simulink model "sampleModel128"  (R2021b)
settings: Solver=VariableStepAuto  StartTime=0.0  StopTime=10.0  RelTol=1e-3
undefined symbols (not defined in the file or in its folder): DiscIntNeverNeededParam
libraries: simulink x5
settings Model: Creator=user  LastModifiedBy=user

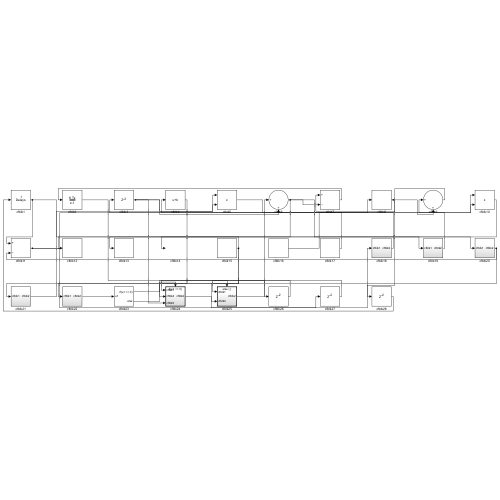
[thumbnail: Simulink's stored preview of the top-level diagram]
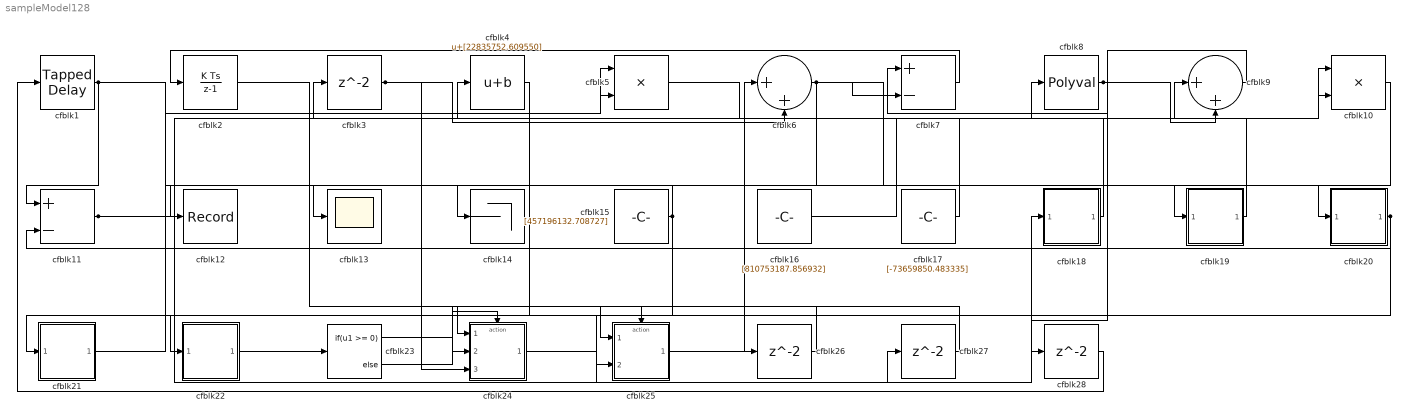
== system sampleModel128 ==
  cfblk1 : simulink/Discrete/Tapped Delay  vinit=0.0  samptime=-1  NumDelays=1  DelayOrder=Oldest  includeCurrent=off
  cfblk10 : Product
  cfblk11 : Sum  Inputs=+-
  cfblk12 : Record  FileSettingsInternal="{\"entries\":[{\"content\":{\"excelSettings\":{\"content\":{},\"type\":\"Streamout.ExcelSettings\"}},\"type\":\"Streamout.FileSettingStorage\",\"uuid\":\"2ee2df8a-bed9-40f4-b3a0-bfcae6ee6a80\"}],\"packageUris\":[\"http://schema.mathworks.com/mf0/streamout_blocks/R2020a\"],\"version\":\"1.0\"}"  SignalsInternal="{\"entries\":[{\"content\":{\"signals\":[{\"content\":{\"blockPath\":[\"sampleModel128/cfblk12\"],\"channel\":[],\"dimensions\":[1],\"domain\":\"sampleModel128/cfblk12\",\"lineColor\":\"#d95319\",\"plots\":[1],\"port\":1,\"sid\":[\"\"],\"signalID\":4493,\"signalName\":\"cfblk15\"},\"type\":\"RecordBlkView.Signal\",\"uuid\":\"ba46f971-64eb-44ee-afbc-2cea7536df18\"}]},\"type\":\"RecordBlkView.InputSignals\",\"uuid\":\"a7605b22-abf8-4e14-8f6f-fc0fcd95ef32\"}],\"packageUris\":[\"http://schema.mathworks.com/mf0/streamout_blocks/R2020a\"],\"version\":\"1.0\"}"  VisualizationBindings="{\"sparklinesplugin\":{\"info\":[{\"bindingParametersList\":[],\"subplotID\":1}]}}"
  cfblk13 : Scope
  cfblk14 : Terminator
  cfblk15 : Constant  Value=[457196132.708727]  SampleTime=1
  cfblk16 : Constant  Value=[810753187.856932]  SampleTime=1
  cfblk17 : Constant  Value=[-73659850.483335]  SampleTime=1
  cfblk18 : Subsystem
  cfblk19 : Subsystem
  cfblk2 : DiscreteIntegrator  ICPrevOutput=DiscIntNeverNeededParam  ICPrevScaledInput=DiscIntNeverNeededParam
  cfblk20 : Subsystem
  cfblk21 : Subsystem
  cfblk22 : Subsystem
  cfblk23 : If  IfExpression=u1 >= 0  SampleTime=1
  cfblk24 : Subsystem  TreatAsAtomicUnit=on
  cfblk25 : Subsystem  TreatAsAtomicUnit=on
  cfblk{3,26..28} (4 alike) : Delay  SampleTime=1
  cfblk4 : Bias  Bias=[22835752.609550]
  cfblk5 : Product
  cfblk6 : Sum  Inputs=|++
  cfblk7 : Sum  Inputs=+-
  cfblk8 : Polyval  Coefs=[ +2.081618890e-019, -1.441693666e-014, +4.719686976e-010, -8.536869453e-006, +1.621573104e-001, -8.087801117e+001 ]
  cfblk9 : Sum  Inputs=|++
  wires:
  cfblk10/1 -> cfblk13/1
  cfblk7/1 -> cfblk2/1
  cfblk11/1 -> cfblk18/1(cfblk1), cfblk8/1
  cfblk15/1 -> cfblk22/1(cfblk1), cfblk24/2(cfblk4), cfblk12/1
  cfblk22/1(cfblk2) -> cfblk23/1
  cfblk16/1 -> cfblk10/1
  cfblk18/1(cfblk2) -> cfblk4/1
  cfblk25/1(cfblk2) -> cfblk6/1
  cfblk20/1(cfblk2) -> cfblk25/2(cfblk4), cfblk11/2
  cfblk5/1 -> cfblk10/2
  cfblk1/1 -> cfblk20/1(cfblk1), cfblk11/1
  cfblk17/1 -> cfblk3/1
  cfblk21/1(cfblk2) -> cfblk5/1
  cfblk8/1 -> cfblk9/2, cfblk28/1
  cfblk6/1 -> cfblk14/1, cfblk7/2, cfblk19/1(cfblk1)
  cfblk4/1 -> cfblk21/1(cfblk1)
  cfblk3/1 -> cfblk5/2, cfblk6/2, cfblk24/3(cfblk5)
  cfblk19/1(cfblk2) -> cfblk9/1
  cfblk9/1 -> cfblk7/1
  cfblk23/1 -> cfblk24/Action
  cfblk23/2 -> cfblk25/Action
  cfblk2/1 -> cfblk26/1
  cfblk26/1 -> cfblk24/1(cfblk1)
  cfblk24/1(cfblk2) -> cfblk27/1
  cfblk27/1 -> cfblk25/1(cfblk1)
  cfblk28/1 -> cfblk1/1

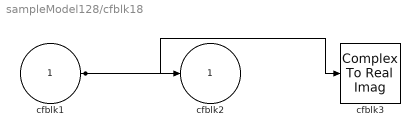
== system sampleModel128/cfblk18 ==
  cfblk1 : Inport
  cfblk3 : ComplexToRealImag
  cfblk2 : Outport
  wires:
  cfblk1/1 -> cfblk2/1, cfblk3/1

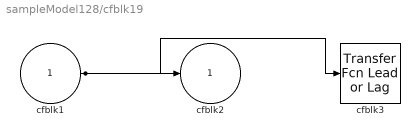
== system sampleModel128/cfblk19 ==
  cfblk1 : Inport
  cfblk3 : simulink/Discrete/Transfer Fcn Lead or Lag  PoleZ=0.95  ZeroZ=0.75  ICPrevOutput=0.0  ICPrevInput=0.0  DoSatur=off
      settings: SourceProductBaseCode=SL
  cfblk2 : Outport
  wires:
  cfblk1/1 -> cfblk2/1, cfblk3/1

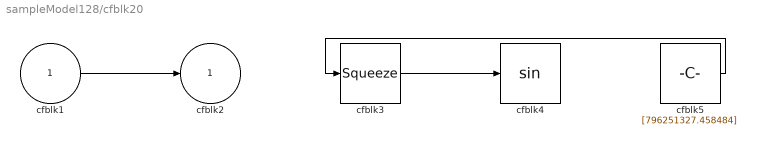
== system sampleModel128/cfblk20 ==
  cfblk1 : Inport
  cfblk3 : Squeeze
  cfblk4 : Trigonometry
  cfblk5 : Constant  Value=[796251327.458484]  SampleTime=1
  cfblk2 : Outport
  wires:
  cfblk1/1 -> cfblk2/1
  cfblk5/1 -> cfblk3/1
  cfblk3/1 -> cfblk4/1

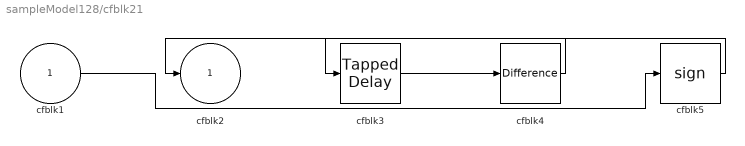
== system sampleModel128/cfblk21 ==
  cfblk1 : Inport
  cfblk3 : simulink/Discrete/Tapped Delay  vinit=0.0  samptime=-1  NumDelays=1  DelayOrder=Oldest  includeCurrent=off
  cfblk4 : simulink/Discrete/Difference  ICPrevInput=0.0  OutMin=[]  OutMax=[]  OutDataTypeStr=Inherit: Inherit via back propagation  OutDataType=fixdt(1, 16)  OutScaling=2^-10  DoSatur=off
  cfblk5 : Signum
  cfblk2 : Outport
  wires:
  cfblk4/1 -> cfblk2/1
  cfblk3/1 -> cfblk4/1
  cfblk1/1 -> cfblk5/1
  cfblk5/1 -> cfblk3/1

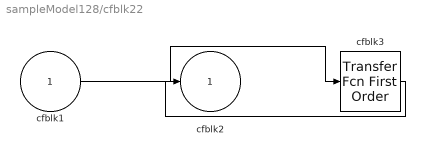
== system sampleModel128/cfblk22 ==
  cfblk1 : Inport
  cfblk3 : simulink/Discrete/Transfer Fcn First Order  PoleZ=0.95  ICPrevOutput=0.0  DoSatur=off
  cfblk2 : Outport
  wires:
  cfblk1/1 -> cfblk3/1
  cfblk3/1 -> cfblk2/1

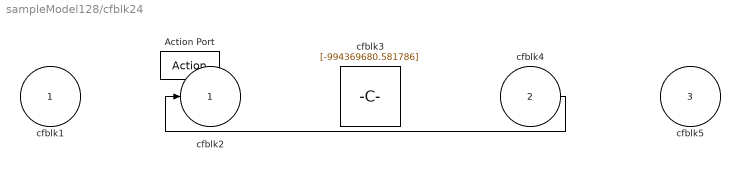
== system sampleModel128/cfblk24 ==
  cfblk1 : Inport
  cfblk4 : Inport  Port=2
  cfblk5 : Inport  Port=3
  Action Port : ActionPort  ActionPortLabel=if(u1 >= 0)
  cfblk3 : Constant  Value=[-994369680.581786]  SampleTime=1
  cfblk2 : Outport
  wires:
  cfblk4/1 -> cfblk2/1

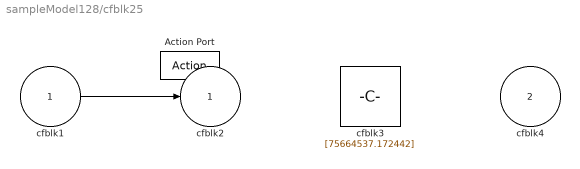
== system sampleModel128/cfblk25 ==
  cfblk1 : Inport
  cfblk4 : Inport  Port=2
  Action Port : ActionPort  ActionPortLabel=else
  cfblk3 : Constant  Value=[75664537.172442]  SampleTime=1
  cfblk2 : Outport
  wires:
  cfblk1/1 -> cfblk2/1
